simulink model "deneme_lineer_003"  (R2020b)
settings: Solver=VariableStepAuto  StartTime=0.0  StopTime=200  RelTol=1e-3
values from neighbouring files (symbols this model uses):
  h0 = 580    [RCAM_initialization.m]
  x0 = [85; 0; 0; 0; 0; 0; 0; 0; 0; xini; yini; h0]    [RCAM_initialization.m]
  xini = 0    [RCAM_initialization.m]
  yini = 0    [RCAM_initialization.m]
undefined symbols (not defined in the file or in its folder): A, B, C, D, RCAM_MODEL_2, u0
libraries: sharedtransform x1
settings Model: Creator=Yigit  LastModifiedBy=Yigit

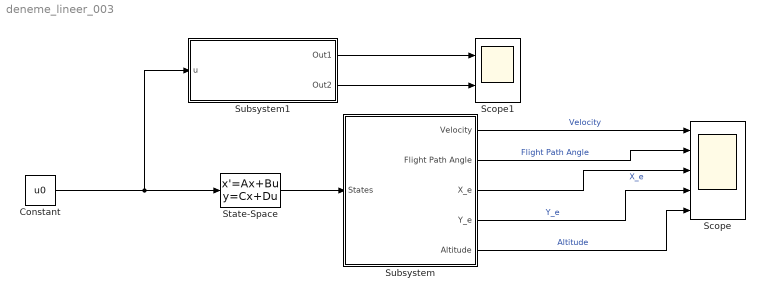
== system deneme_lineer_003 ==
  Constant : Constant  Value=u0
  Scope : Scope  NumInputPorts=5
  Scope1 : Scope  NumInputPorts=2
  State-Space : StateSpace  A=A  B=B  C=C  D=D  InitialCondition=x0
  Subsystem : Subsystem
  Subsystem1 : Subsystem
  wires:
  State-Space/1 -> Subsystem/1(States)
  Subsystem/1(Velocity) -> Scope/1  "Velocity"
  Subsystem/2(Flight Path Angle) -> Scope/2  "Flight Path Angle"
  Subsystem/4(Y_e) -> Scope/4  "Y_e"
  Subsystem/3(X_e) -> Scope/3  "X_e"
  Subsystem/5(Altitude) -> Scope/5  "Altitude"
  Subsystem1/1(Out1) -> Scope1/1
  Subsystem1/2(Out2) -> Scope1/2
  Constant/1 -> State-Space/1, Subsystem1/1(u)

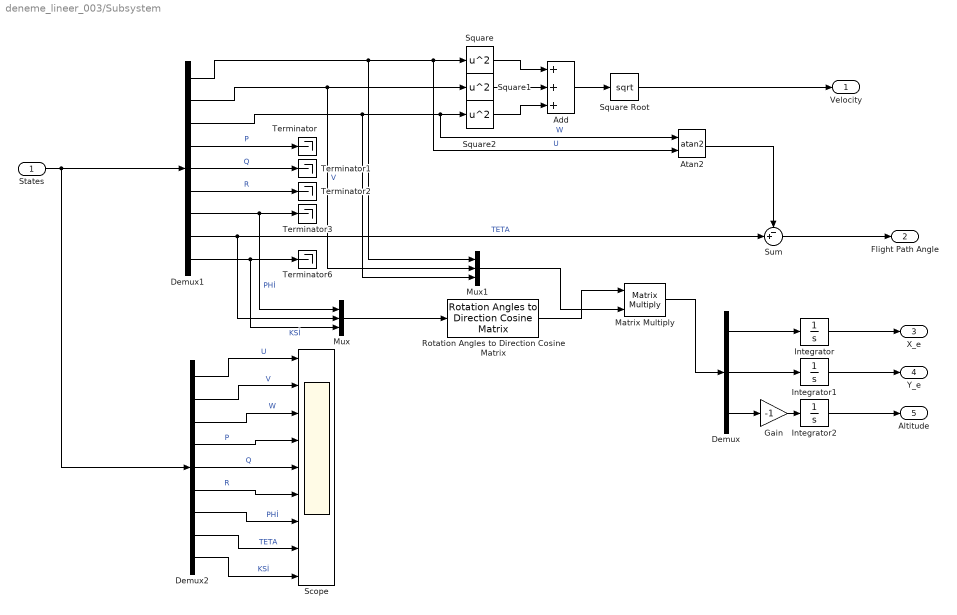
== system deneme_lineer_003/Subsystem ==
  States : Inport
  Add : Sum  Inputs=+++
  Atan2 : Trigonometry  Operator=atan2
  Demux : Demux  Outputs=3
  Demux1 : Demux  Outputs=9
  Demux2 : Demux  Outputs=9
  Gain : Gain  Gain=-1
  Integrator : Integrator  InitialCondition=xini
  Integrator1 : Integrator  InitialCondition=yini
  Integrator2 : Integrator  InitialCondition=h0
  Matrix Multiply : Product  Multiplication=Matrix(*)
  Mux : Mux  Inputs=3
  Mux1 : Mux  Inputs=3
  Rotation Angles to Direction Cosine Matrix : sharedtransform/Rotation Angles to Direction Cosine Matrix  rotationOrder=ZYX  aMode=aMode
      settings: SourceProductBaseCode=AE,PW,MT,UV,VE,VP
  Scope : Scope  NumInputPorts=9
  Square : Math  Operator=square  SaturateOnIntegerOverflow=on
  Square Root : Sqrt  SaturateOnIntegerOverflow=on
  Square1 : Math  Operator=square  SaturateOnIntegerOverflow=on
  Square2 : Math  Operator=square  SaturateOnIntegerOverflow=on
  Sum : Sum  Inputs=-+|
  Terminator{,1..3,6} (5 alike) : Terminator
  Velocity : Outport
  Flight Path Angle : Outport  Port=2
  X_e : Outport  Port=3
  Y_e : Outport  Port=4
  Altitude : Outport  Port=5
  wires:
  Demux1/1 -> Mux1/1, Square/1, Atan2/2  "U"
  Demux1/4 -> Terminator/1  "P"
  Demux1/9 -> Mux/3, Terminator6/1  "KSİ"
  Demux1/7 -> Mux/1, Terminator3/1  "PHİ"
  Square Root/1 -> Velocity/1
  Add/1 -> Square Root/1
  Square1/1 -> Add/2
  Sum/1 -> Flight Path Angle/1
  Atan2/1 -> Sum/1
  Demux1/6 -> Terminator2/1  "R"
  Demux1/5 -> Terminator1/1  "Q"
  Demux1/2 -> Mux1/2, Square1/1  "V"
  Square/1 -> Add/1
  Demux1/8 -> Mux/2, Sum/2  "TETA"
  Demux1/3 -> Mux1/3, Atan2/1, Square2/1  "W"
  Square2/1 -> Add/3
  Mux/1 -> Rotation Angles to Direction Cosine Matrix/1
  Rotation Angles to Direction Cosine Matrix/1 -> Matrix Multiply/1
  Mux1/1 -> Matrix Multiply/2
  Matrix Multiply/1 -> Demux/1
  Demux/1 -> Integrator/1
  Demux/2 -> Integrator1/1
  Demux/3 -> Gain/1
  Gain/1 -> Integrator2/1
  Integrator/1 -> X_e/1
  Integrator1/1 -> Y_e/1
  Integrator2/1 -> Altitude/1
  States/1 -> Demux2/1, Demux1/1
  Demux2/5 -> Scope/5  "Q"
  Demux2/4 -> Scope/4  "P"
  Demux2/6 -> Scope/6  "R"
  Demux2/3 -> Scope/3  "W"
  Demux2/7 -> Scope/7  "PHİ"
  Demux2/2 -> Scope/2  "V"
  Demux2/8 -> Scope/8  "TETA"
  Demux2/1 -> Scope/1  "U"
  Demux2/9 -> Scope/9  "KSİ"

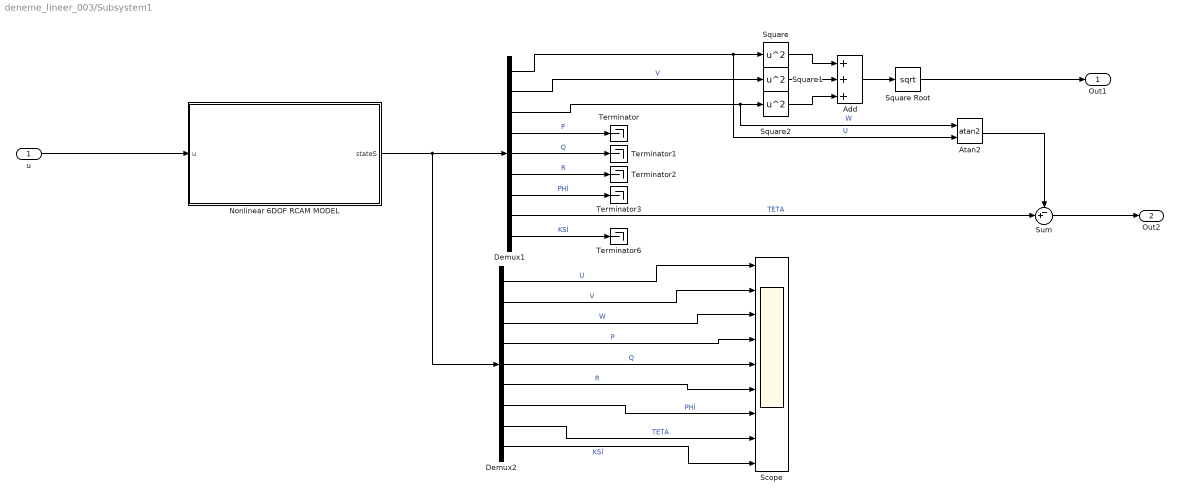
== system deneme_lineer_003/Subsystem1 ==
  u : Inport
  Add : Sum  Inputs=+++
  Atan2 : Trigonometry  Operator=atan2
  Demux1 : Demux  Outputs=9
  Demux2 : Demux  Outputs=9
  Nonlinear 6DOF RCAM MODEL : Subsystem
  Scope : Scope  NumInputPorts=9
  Square : Math  Operator=square  SaturateOnIntegerOverflow=on
  Square Root : Sqrt  SaturateOnIntegerOverflow=on
  Square1 : Math  Operator=square  SaturateOnIntegerOverflow=on
  Square2 : Math  Operator=square  SaturateOnIntegerOverflow=on
  Sum : Sum  Inputs=-+|
  Terminator{,1..3,6} (5 alike) : Terminator
  Out1 : Outport
  Out2 : Outport  Port=2
  wires:
  Square2/1 -> Add/3
  Demux1/4 -> Terminator/1  "P"
  Add/1 -> Square Root/1
  Demux1/5 -> Terminator1/1  "Q"
  Demux1/1 -> Square/1, Atan2/2  "U"
  Demux1/3 -> Atan2/1, Square2/1  "W"
  Demux1/8 -> Sum/2  "TETA"
  Demux1/6 -> Terminator2/1  "R"
  Square Root/1 -> Out1/1
  Square/1 -> Add/1
  Demux1/9 -> Terminator6/1  "KSİ"
  Demux1/2 -> Square1/1  "V"
  Square1/1 -> Add/2
  u/1 -> Nonlinear 6DOF RCAM MODEL/1(u)
  Atan2/1 -> Sum/1
  Sum/1 -> Out2/1
  Demux1/7 -> Terminator3/1  "PHİ"
  Demux2/9 -> Scope/9  "KSİ"
  Demux2/1 -> Scope/1  "U"
  Demux2/8 -> Scope/8  "TETA"
  Demux2/6 -> Scope/6  "R"
  Demux2/5 -> Scope/5  "Q"
  Demux2/4 -> Scope/4  "P"
  Demux2/3 -> Scope/3  "W"
  Demux2/7 -> Scope/7  "PHİ"
  Nonlinear 6DOF RCAM MODEL/1(stateS) -> Demux2/1, Demux1/1
  Demux2/2 -> Scope/2  "V"

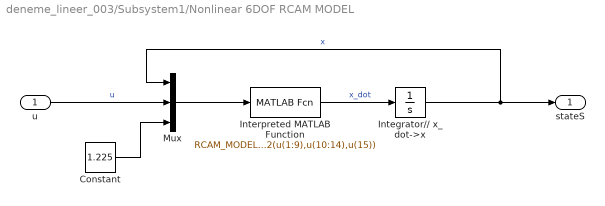
== system deneme_lineer_003/Subsystem1/Nonlinear 6DOF RCAM MODEL ==
  u : Inport
  Constant : Constant  Value=1.225
  Integrator// x_dot->x : Integrator  InitialCondition=x0
  Interpreted MATLAB Function : MATLABFcn  MATLABFcn=RCAM_MODEL_2(u(1:9),u(10:14),u(15))
  Mux : Mux  Inputs=3
  stateS : Outport
  wires:
  Interpreted MATLAB Function/1 -> Integrator// x_dot->x/1  "x_dot"
  Mux/1 -> Interpreted MATLAB Function/1
  Integrator// x_dot->x/1 -> stateS/1, Mux/1  "x"
  Constant/1 -> Mux/3
  u/1 -> Mux/2  "u"
